simulink model "test_sin"  (R2022a)
settings: Solver=VariableStepAuto  StartTime=0  StopTime=10  FixedStep=0.1  MaxStep=0.01  RelTol=1e-3
model workspace (MAT data in the model file):
  Kdbf = 5
  Kdmf = [2  0  0  0; 0  2  0  0; 0  0  2  0; 0  0  0  2]
  Kibc = 0.5
  Kimc = [0.6  0  0  0; 0  0.5  0  0; 0  0  0.4  0; 0  0  0  0.5]
  Kimf = [2  0  0  0; 0  2  0  0; 0  0  2  0; 0  0  0  2]
  Kpbc = 1
  Kpbf = 0.1
  Kpmc = [2  0  0  0; 0  2  0  0; 0  0  2  0; 0  0  0  2]
  Kpmf = [0.1  0  0  0; 0  0.1  0  0; 0  0  0.1  0; 0  0  0  0.1]
  dq0 = 0
  dqm = [0; 0; 0; 0]
  q0 = 0.3
  q0_d = 0
  qm = [0.1; 0.15; 0.25; 0.3]
  qm_d = [0; 0; 0; 0]
settings Model: Creator=43840  LastModifiedBy=43840

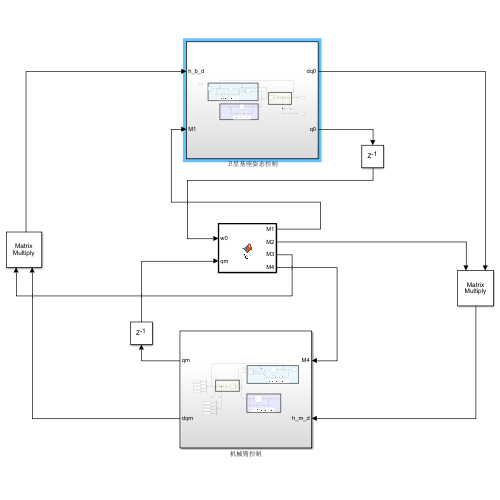
[thumbnail: Simulink's stored preview of the top-level diagram]
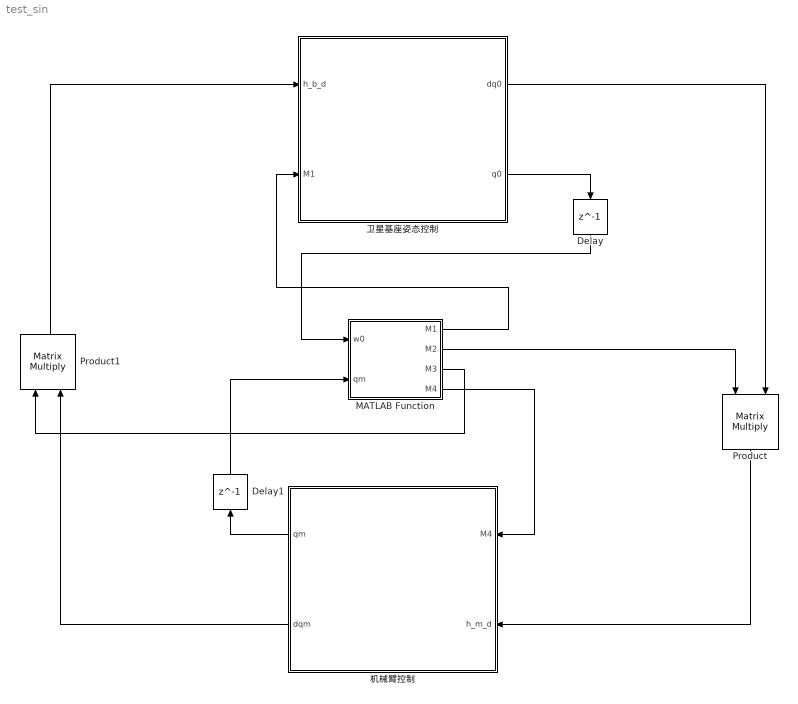
== system test_sin ==
  Delay : Delay  DelayLength=1
  Delay1 : Delay  DelayLength=1
  MATLAB Function : MATLAB Function  TreatAsAtomicUnit=on
  Product : Product  Multiplication=Matrix(*)
  Product1 : Product  Multiplication=Matrix(*)
  卫星基座姿态控制 : Subsystem
  机械臂控制 : Subsystem
  wires:
  Product1/1 -> 卫星基座姿态控制/1(h_b_d)
  机械臂控制/2(dqm) -> Product1/2
  Product/1 -> 机械臂控制/2(h_m_d)
  卫星基座姿态控制/1(dq0) -> Product/2
  机械臂控制/1(qm) -> Delay1/1
  卫星基座姿态控制/2(q0) -> Delay/1
  MATLAB Function/1(M1) -> 卫星基座姿态控制/2(M1)
  MATLAB Function/4(M4) -> 机械臂控制/1(M4)
  MATLAB Function/2(M2) -> Product/1
  MATLAB Function/3(M3) -> Product1/1
  Delay/1 -> MATLAB Function/1(w0)
  Delay1/1 -> MATLAB Function/2(qm)

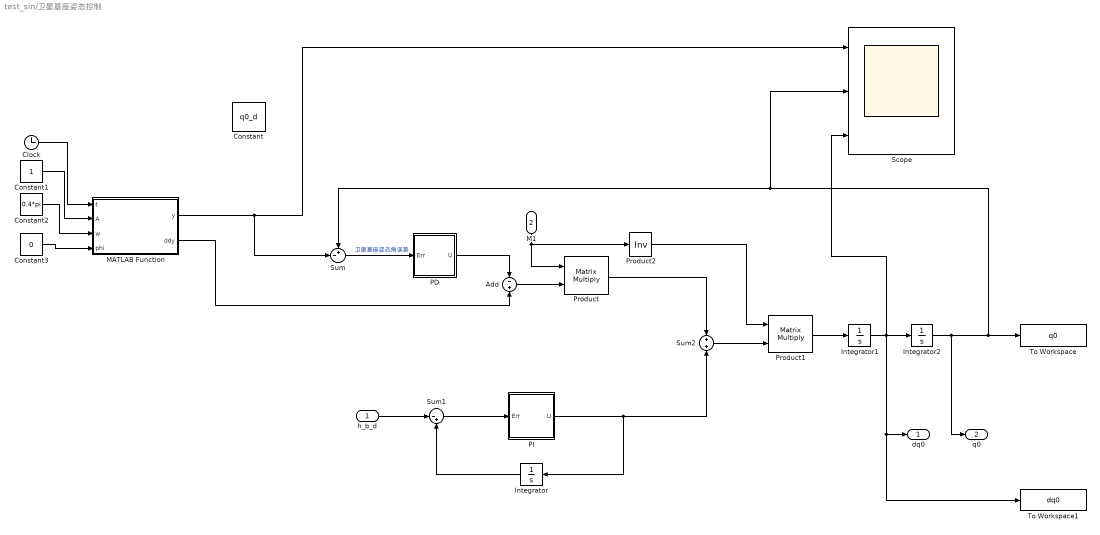
== system test_sin/卫星基座姿态控制 ==
  h_b_d : Inport
  M1 : Inport  Port=2
  Add : Sum  Inputs=-+
  Clock : Clock
  Constant : Constant  Value=q0_d  VectorParams1D=off
  Constant1 : Constant
  Constant2 : Constant  Value=0.4*pi
  Constant3 : Constant  Value=0
  Integrator : Integrator
  Integrator1 : Integrator  InitialCondition=dq0
  Integrator2 : Integrator  InitialCondition=q0
  MATLAB Function : MATLAB Function  TreatAsAtomicUnit=on
  PD : Subsystem
  PI : Subsystem
  Product : Product  Multiplication=Matrix(*)
  Product1 : Product  Multiplication=Matrix(*)
  Product2 : Product  Inputs=/  Multiplication=Matrix(*)
  Scope : Scope  NumInputPorts=3
  Sum : Sum  Inputs=+-|
  Sum1 : Sum  Inputs=|-+
  Sum2 : Sum  Inputs=+|+
  To Workspace : ToWorkspace  VariableName=q0  SampleTime=-1
      settings: Save2DSignal=2-D array (concatenate along first dimension)
  To Workspace1 : ToWorkspace  VariableName=dq0  SampleTime=-1
      settings: Save2DSignal=2-D array (concatenate along first dimension)
  dq0 : Outport
  q0 : Outport  Port=2
  wires:
  Sum/1 -> PD/1(Err)  "卫星基座姿态角误差"
  Integrator/1 -> Sum1/2
  Sum1/1 -> PI/1(Err)
  Product/1 -> Sum2/1
  PD/1(U) -> Add/1
  Add/1 -> Product/2
  PI/1(U) -> Sum2/2, Integrator/1
  h_b_d/1 -> Sum1/1
  Integrator1/1 -> To Workspace1/1, dq0/1, Scope/3, Integrator2/1
  Integrator2/1 -> q0/1, To Workspace/1, Scope/2, Sum/1
  M1/1 -> Product2/1, Product/1
  Product2/1 -> Product1/1
  Product1/1 -> Integrator1/1
  Sum2/1 -> Product1/2
  MATLAB Function/2(ddy) -> Add/2
  MATLAB Function/1(y) -> Scope/1, Sum/2
  Constant3/1 -> MATLAB Function/4(phi)
  Constant2/1 -> MATLAB Function/3(w)
  Clock/1 -> MATLAB Function/1(t)
  Constant1/1 -> MATLAB Function/2(A)

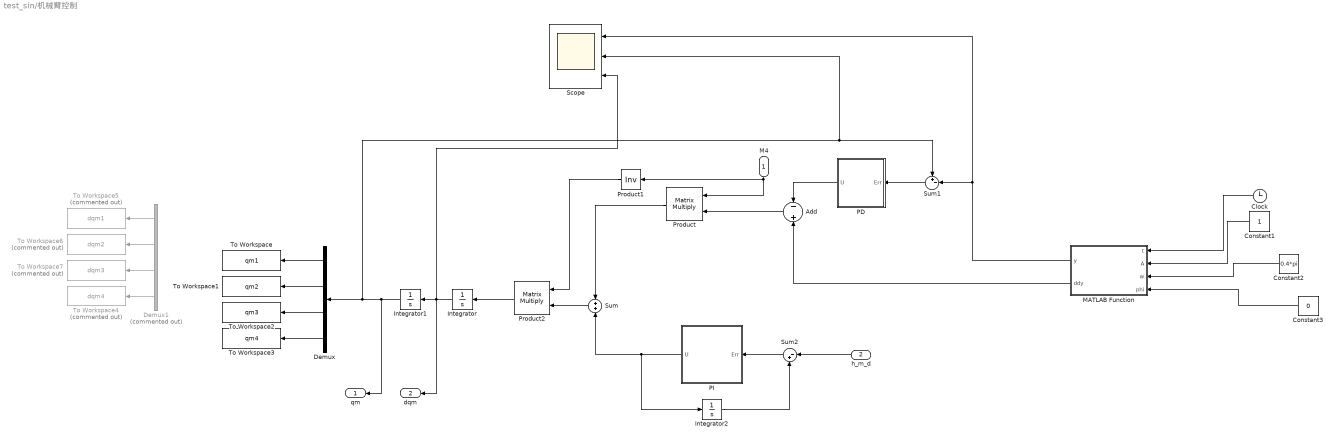
== system test_sin/机械臂控制 ==
  M4 : Inport
  h_m_d : Inport  Port=2
  Add : Sum  Inputs=-+
  Clock : Clock
  Constant1 : Constant
  Constant2 : Constant  Value=0.4*pi
  Constant3 : Constant  Value=0
  Demux : Demux
  Demux1 : Demux  Commented=on
  Integrator : Integrator  InitialCondition=dqm
  Integrator1 : Integrator  InitialCondition=qm
  Integrator2 : Integrator
  MATLAB Function : MATLAB Function  TreatAsAtomicUnit=on
  PD : Subsystem
  PI : Subsystem
  Product : Product  Multiplication=Matrix(*)
  Product1 : Product  Inputs=/  Multiplication=Matrix(*)
  Product2 : Product  Multiplication=Matrix(*)
  Scope : Scope  NumInputPorts=3
  Sum : Sum
  Sum1 : Sum  Inputs=+-|
  Sum2 : Sum  Inputs=|-+
  To Workspace : ToWorkspace  VariableName=qm1  SampleTime=-1
      settings: Save2DSignal=2-D array (concatenate along first dimension)
  To Workspace1 : ToWorkspace  VariableName=qm2  SampleTime=-1
      settings: Save2DSignal=2-D array (concatenate along first dimension)
  To Workspace2 : ToWorkspace  VariableName=qm3  SampleTime=-1
      settings: Save2DSignal=2-D array (concatenate along first dimension)
  To Workspace3 : ToWorkspace  VariableName=qm4  SampleTime=-1
      settings: Save2DSignal=2-D array (concatenate along first dimension)
  To Workspace4 : ToWorkspace  Commented=on  VariableName=dqm4  SampleTime=-1
      settings: Save2DSignal=2-D array (concatenate along first dimension)
  To Workspace5 : ToWorkspace  Commented=on  VariableName=dqm1  SampleTime=-1
      settings: Save2DSignal=2-D array (concatenate along first dimension)
  To Workspace6 : ToWorkspace  Commented=on  VariableName=dqm2  SampleTime=-1
      settings: Save2DSignal=2-D array (concatenate along first dimension)
  To Workspace7 : ToWorkspace  Commented=on  VariableName=dqm3  SampleTime=-1
      settings: Save2DSignal=2-D array (concatenate along first dimension)
  qm : Outport
  dqm : Outport  Port=2
  wires:
  Integrator2/1 -> Sum2/2
  PI/1(U) -> Sum/2, Integrator2/1
  Sum2/1 -> PI/1(Err)
  Product2/1 -> Integrator/1
  Sum1/1 -> PD/1(Err)
  Product/1 -> Sum/1
  Add/1 -> Product/2
  PD/1(U) -> Add/1
  h_m_d/1 -> Sum2/1
  Demux/1 -> To Workspace/1
  Demux/2 -> To Workspace1/1
  Demux/3 -> To Workspace2/1
  Demux/4 -> To Workspace3/1
  M4/1 -> Product/1, Product1/1
  Integrator/1 -> dqm/1, Scope/3, Integrator1/1
  Demux1/1 -> To Workspace5/1
  Demux1/2 -> To Workspace6/1
  Demux1/3 -> To Workspace7/1
  Demux1/4 -> To Workspace4/1
  Product1/1 -> Product2/1
  Integrator1/1 -> qm/1, Demux/1, Scope/2, Sum1/1
  Sum/1 -> Product2/2
  Constant2/1 -> MATLAB Function/3(w)
  Constant3/1 -> MATLAB Function/4(phi)
  Clock/1 -> MATLAB Function/1(t)
  Constant1/1 -> MATLAB Function/2(A)
  MATLAB Function/1(y) -> Scope/1, Sum1/2
  MATLAB Function/2(ddy) -> Add/2

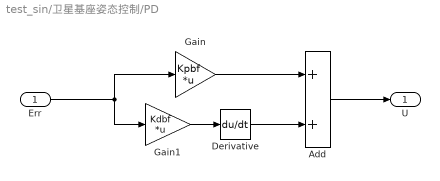
== system test_sin/卫星基座姿态控制/PD ==
  Err : Inport
  Add : Sum
  Derivative : Derivative
  Gain : Gain  Gain=Kpbf  Multiplication=Matrix(K*u)
  Gain1 : Gain  Gain=Kdbf  Multiplication=Matrix(K*u)
  U : Outport
  wires:
  Err/1 -> Gain1/1, Gain/1
  Gain1/1 -> Derivative/1
  Gain/1 -> Add/1
  Derivative/1 -> Add/2
  Add/1 -> U/1

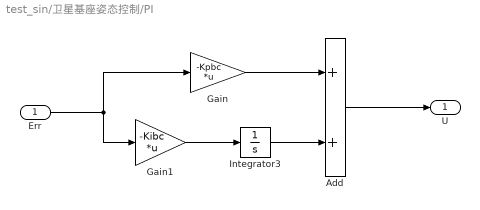
== system test_sin/卫星基座姿态控制/PI ==
  Err : Inport
  Add : Sum
  Gain : Gain  Gain=-Kpbc  Multiplication=Matrix(K*u)
  Gain1 : Gain  Gain=-Kibc  Multiplication=Matrix(K*u)
  Integrator3 : Integrator
  U : Outport
  wires:
  Gain1/1 -> Integrator3/1
  Add/1 -> U/1
  Gain/1 -> Add/1
  Err/1 -> Gain1/1, Gain/1
  Integrator3/1 -> Add/2

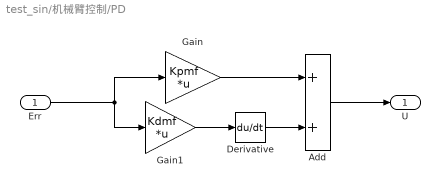
== system test_sin/机械臂控制/PD ==
  Err : Inport
  Add : Sum
  Derivative : Derivative
  Gain : Gain  Gain=Kpmf  Multiplication=Matrix(K*u)
  Gain1 : Gain  Gain=Kdmf  Multiplication=Matrix(K*u)
  U : Outport
  wires:
  Err/1 -> Gain1/1, Gain/1
  Gain1/1 -> Derivative/1
  Gain/1 -> Add/1
  Derivative/1 -> Add/2
  Add/1 -> U/1

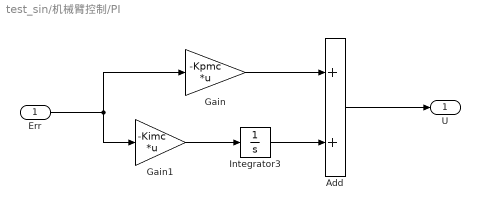
== system test_sin/机械臂控制/PI ==
  Err : Inport
  Add : Sum
  Gain : Gain  Gain=-Kpmc  Multiplication=Matrix(K*u)
  Gain1 : Gain  Gain=-Kimc  Multiplication=Matrix(K*u)
  Integrator3 : Integrator
  U : Outport
  wires:
  Gain1/1 -> Integrator3/1
  Add/1 -> U/1
  Gain/1 -> Add/1
  Err/1 -> Gain1/1, Gain/1
  Integrator3/1 -> Add/2

== matlab function test_sin/卫星基座姿态控制/MATLAB Function ==
  data: t input; y output; A input; w input; phi input; ddy output
function [y, ddy] = fcn(t,A,w,phi)

y=0;
% dy=0;
ddy=0;

y = A*sin(w*t+phi);
% dy=A*w*cos(w*t+phi);
ddy=-A*w*w*sin(w*t+phi);

== matlab function test_sin/MATLAB Function ==
  data: w0 input; M1 output; qm input; M2 output; M3 output; M4 output
function [M1, M2, M3, M4] = fcn(w0,qm)

coder.extrinsic("calc_Mass")

M1=zeros(1,1);
M2=zeros(4,1);
M3=zeros(1,4);
M4=zeros(4,4);

[M1, M2, M3, M4]=calc_Mass(w0,qm);

== matlab function test_sin/机械臂控制/MATLAB Function ==
  data: t input; y output; A input; w input; phi input; ddy output
function [y, ddy] = fcn(t,A,w,phi)

y=zeros(4,1);
% dy=0;
ddy=zeros(4,1);

y = [A*sin(w*t+phi);A*sin(w*t+phi);A*sin(w*t+phi);A*sin(w*t+phi)];
% dy=A*w*cos(w*t+phi);
ddy=[-A*w*w*sin(w*t+phi);-A*w*w*sin(w*t+phi);-A*w*w*sin(w*t+phi);-A*w*w*sin(w*t+phi)];
